simulink model "Actuating_lab1_2_2016b"  (R2016b)
settings: Solver=VariableStepAuto  StartTime=0.0  StopTime=20  RelTol=1e-3
libraries: simulink_extras x1, simulink x1
settings Model: Creator=kamzab95  LastModifiedBy=kamzab95

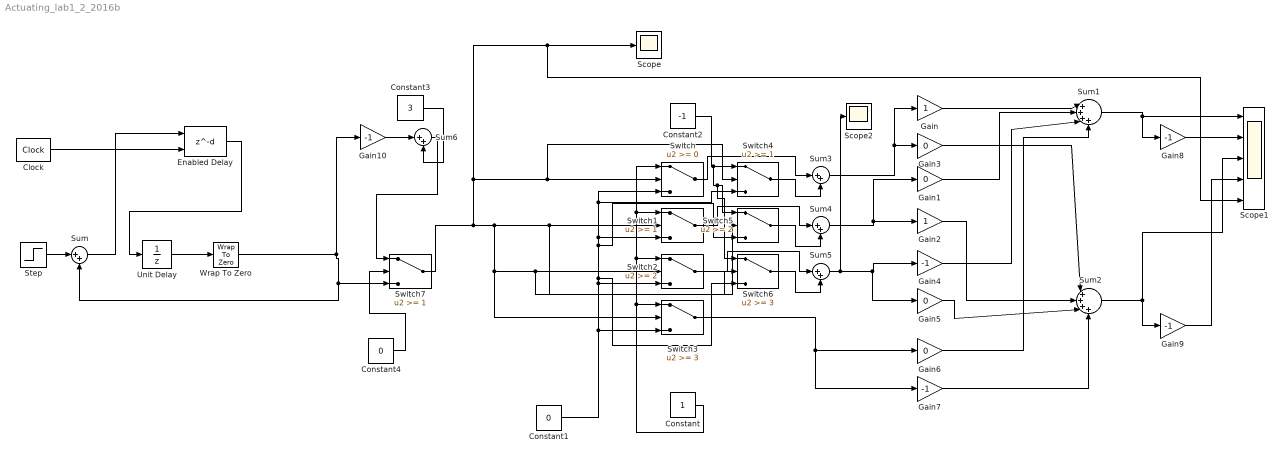
== system Actuating_lab1_2_2016b ==
  Clock : simulink_extras/Flip Flops/Clock  period=4
  Constant : Constant
  Constant1 : Constant  Value=0
  Constant2 : Constant  Value=-1
  Constant3 : Constant  Value=3
  Constant4 : Constant  Value=0
  Enabled Delay : Delay  DelayLengthSource=Input port
      settings: InputPortMap=u0,p1
  Gain : Gain
  Gain{1,3,5..6} (4 alike) : Gain  Gain=0
  Gain{4,7..10} (5 alike) : Gain  Gain=-1
  Gain2 : Gain
  Scope : Scope
  Scope1 : Scope  NumInputPorts=5
  Scope2 : Scope
  Step : Step  SampleTime=0
  Sum{,3..6} (5 alike) : Sum  Inputs=|++
  Sum1 : Sum  Inputs=|++++
  Sum2 : Sum  Inputs=|++++
  Switch : Switch
  Switch1 : Switch  Threshold=1
  Switch2 : Switch  Threshold=2
  Switch3 : Switch  Threshold=3
  Switch4 : Switch  Threshold=1
  Switch5 : Switch  Threshold=2
  Switch6 : Switch  Threshold=3
  Switch7 : Switch  Threshold=1
  Unit Delay : UnitDelay  SampleTime=-1
  Wrap To Zero : simulink/Discontinuities/Wrap To Zero  Threshold=3
  wires:
  Step/1 -> Sum/1
  Unit Delay/1 -> Wrap To Zero/1
  Wrap To Zero/1 -> Sum/2, Switch7/3, Gain10/1
  Gain/1 -> Sum1/1
  Gain1/1 -> Sum1/2
  Gain4/1 -> Sum1/3
  Gain6/1 -> Sum1/4
  Gain3/1 -> Sum2/1
  Gain2/1 -> Sum2/2
  Gain5/1 -> Sum2/3
  Gain7/1 -> Sum2/4
  Sum1/1 -> Gain8/1, Scope1/1
  Sum2/1 -> Scope1/3, Gain9/1
  Constant/1 -> Switch3/1, Switch2/1, Switch1/1, Switch/1
  Constant1/1 -> Switch6/3, Switch5/3, Switch4/3, Switch/3, Switch1/3, Switch2/3, Switch3/3
  Constant2/1 -> Switch6/1, Switch5/1, Switch4/1
  Switch/1 -> Sum3/1
  Switch4/1 -> Sum3/2
  Sum3/1 -> Gain3/1, Gain/1
  Switch5/1 -> Sum4/2
  Switch1/1 -> Sum4/1
  Switch6/1 -> Sum5/2
  Switch2/1 -> Sum5/1
  Sum4/1 -> Gain2/1, Gain1/1
  Sum5/1 -> Scope2/1, Gain5/1, Gain4/1
  Switch3/1 -> Gain7/1, Gain6/1
  Switch7/1 -> Switch3/2, Switch6/2, Switch2/2, Switch5/2, Switch1/2, Switch4/2, Switch/2, Scope1/5, Scope/1
  Gain10/1 -> Sum6/1
  Constant3/1 -> Sum6/2
  Sum6/1 -> Switch7/1
  Sum/1 -> Enabled Delay/1
  Enabled Delay/1 -> Unit Delay/1
  Clock/1 -> Enabled Delay/2
  Constant4/1 -> Switch7/2
  Gain8/1 -> Scope1/2
  Gain9/1 -> Scope1/4
